simulink model "CarlaRosMatlab_LaneDetection"  (R2019b)
settings: Solver=FixedStepAuto  StartTime=0.0  StopTime=inf  FixedStep=0.2  RelTol=1e-3  EnableMultiTasking=on
model workspace (MAT data in the model file):
  SL_ROS_VariableLengthArrays_MaxSizes.CommonInfo.ArrayTruncateAction = 'EmitWarning'
  SL_ROS_VariableLengthArrays_MaxSizes.MsgTypeMap = containers.Map
  SL_ROS_VariableLengthArrays_MaxSizes.MsgTypeMap.serialization.keys = {'sensor_msgs/CompressedImage', 'sensor_msgs/Image', 'sensor_msgs/PointCloud2'}
  SL_ROS_VariableLengthArrays_MaxSizes.MsgTypeMap.serialization.values{1}(1).PropertyName = 'Format'
  SL_ROS_VariableLengthArrays_MaxSizes.MsgTypeMap.serialization.values{1}(1).DataType = 'uint8'
  SL_ROS_VariableLengthArrays_MaxSizes.MsgTypeMap.serialization.values{1}(1).MaxLength = 128
  SL_ROS_VariableLengthArrays_MaxSizes.MsgTypeMap.serialization.values{1}(2).PropertyName = 'Data'
  SL_ROS_VariableLengthArrays_MaxSizes.MsgTypeMap.serialization.values{1}(2).DataType = 'uint8'
  SL_ROS_VariableLengthArrays_MaxSizes.MsgTypeMap.serialization.values{1}(2).MaxLength = 128000
  SL_ROS_VariableLengthArrays_MaxSizes.MsgTypeMap.serialization.values{2}(1).PropertyName = 'Data'
  SL_ROS_VariableLengthArrays_MaxSizes.MsgTypeMap.serialization.values{2}(1).DataType = 'uint8'
  SL_ROS_VariableLengthArrays_MaxSizes.MsgTypeMap.serialization.values{2}(1).MaxLength = 8294400
  SL_ROS_VariableLengthArrays_MaxSizes.MsgTypeMap.serialization.values{2}(2).PropertyName = 'Encoding'
  SL_ROS_VariableLengthArrays_MaxSizes.MsgTypeMap.serialization.values{2}(2).DataType = 'uint8'
  SL_ROS_VariableLengthArrays_MaxSizes.MsgTypeMap.serialization.values{2}(2).MaxLength = 128
  SL_ROS_VariableLengthArrays_MaxSizes.MsgTypeMap.serialization.values{3}(1).PropertyName = 'Data'
  SL_ROS_VariableLengthArrays_MaxSizes.MsgTypeMap.serialization.values{3}(1).DataType = 'uint8'
  SL_ROS_VariableLengthArrays_MaxSizes.MsgTypeMap.serialization.values{3}(1).MaxLength = 182976
  SL_ROS_VariableLengthArrays_MaxSizes.MsgTypeMap.serialization.values{3}(2).PropertyName = 'Fields'
  SL_ROS_VariableLengthArrays_MaxSizes.MsgTypeMap.serialization.values{3}(2).DataType = 'sensor_msgs/PointField'
  SL_ROS_VariableLengthArrays_MaxSizes.MsgTypeMap.serialization.values{3}(2).MaxLength = 16
  SL_ROS_VariableLengthArrays_MaxSizes.MsgTypeMap.serialization.uniformity = 0
  SL_ROS_VariableLengthArrays_MaxSizes.MsgTypeMap.serialization.keyType = 'char'
  SL_ROS_VariableLengthArrays_MaxSizes.MsgTypeMap.serialization.valueType = 'any'
undefined symbols (not defined in the file or in its folder): Brake, Steer, Throttle
libraries: robotlib x10, visiontextngfix x2, visionsinks x2
settings Model: Creator=sprinkle  LastModifiedBy=aa
settings DataIOCC: ReturnWorkspaceOutputs=off
settings OptimizationCC: LifeSpan=Inf  MaxStackSize=64  EfficientTunableParamExpr=on
settings DebuggingCC: SFUnexpectedBacktrackingDiag=warning  SFNoUnconditionalDefaultTransitionDiag=warning  ArithmeticOperatorsInVariantConditions=warning
settings HardwareCC: ProdBitPerPointer=32  ProdBitPerSizeT=32  ProdBitPerPtrDiffT=32  ProdLargestAtomicFloat=None  ProdIntDivRoundTo=Undefined  ProdEndianess=Unspecified  ProdWordSize=32  ProdHWDeviceType=Generic->Unspecified (assume 32-bit Generic)
settings SFSimCC: SimUseLocalCustomCode=off  MATLABDynamicMemAlloc=off  CustomCodeUndefinedFunction=UseInterfaceOnly
settings RTWCC: SystemTargetFile=ert.tlc  HardwareBoard=Robot Operating System (ROS)  TLCOptions=-aInlineSetEventsForThisBaseRateFcn=TLC_FALSE -aSuppressMultiTaskScheduler=TLC_FALSE -aRateBasedStepFcn=0  TemplateMakefile=ert_default_tmf  GenerateReport=on  RTWUseLocalCustomCode=off  Toolchain=Catkin  IncludeHyperlinkInReport=on  LaunchReport=on  TargetLang=C++  GenerateTraceInfo=on  GenerateTraceReport=on  GenerateTraceReportSl=on  GenerateTraceReportSf=on  GenerateTraceReportEml=on
settings CodeAppCC: ForceParamTrailComments=on  IgnoreCustomStorageClasses=off  OperatorAnnotations=on  SimulinkDataObjDesc=on  SFDataObjDesc=on  MATLABFcnDesc=on  InsertBlockDesc=on  StateflowObjectComments=on  MATLABSourceComments=on
settings ERTTargetCC: MultiwordLength=2048
settings ConfigComp: CovMetricSettings=dw  CovHtmlReporting=on  CovSaveCumulativeToWorkspaceVar=on  CovSaveSingleToWorkspaceVar=on  CovExternalEMLEnable=off

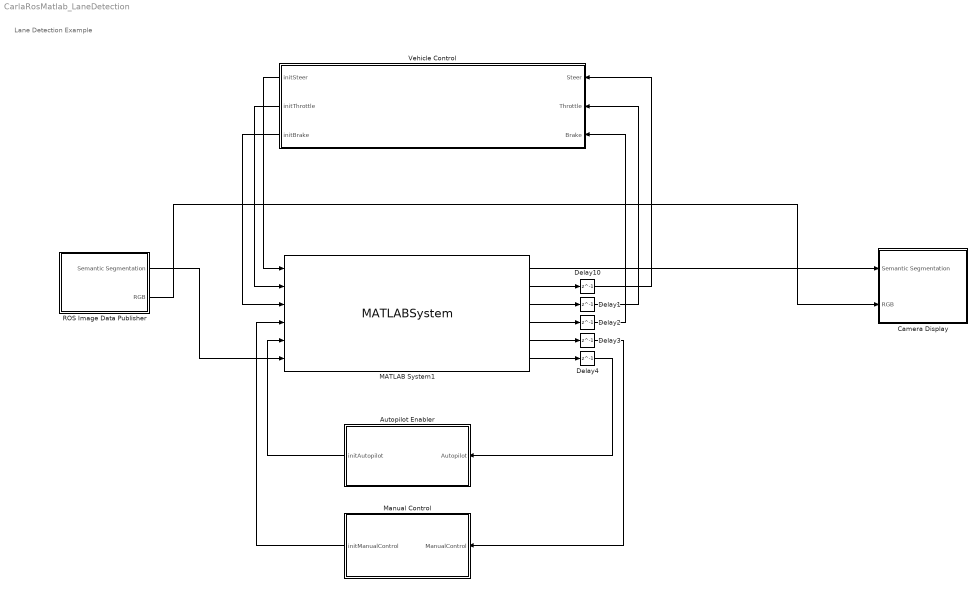
== system CarlaRosMatlab_LaneDetection ==
  note: Lane Detection Example
  Autopilot Enabler : Subsystem
  Camera Display : Subsystem
  Delay{1..4,10} (5 alike) : Delay  DelayLength=1  InitialCondition=0
  MATLAB System1 : MATLABSystem  System=LaneDetection  SimulateUsing=Interpreted execution
      mask Type: LaneDetection
      mask Display:
      | disp('LaneDetection');
      | port_label('input',1,'steer_prev');
      | port_label('input',2,'throttle_prev');
      | port_label('input',3,'brake_prev');
      | port_label('input',4,'manualcontrol_prev');
      | port_label('input',5,'autopilot_prev');
      | port_label('input',6,'SEMANTIC_IN');
      | port_label('output',1,'SEMANTIC_SEGMENTATION');
      | port_label('output',2,'steer');
      | port_label('output',3,'throttle');
      | port_label('output',4,'brake');
      | port_label('output',5,'manualcontrol');
      | port_label('output',6,'autopilot');
  Manual Control : Subsystem
  ROS Image Data Publisher : Subsystem
  Vehicle Control : Subsystem
  wires:
  MATLAB System1/1 -> Camera Display/1(Semantic Segmentation)
  ROS Image Data Publisher/2(RGB) -> Camera Display/2(RGB)
  Autopilot Enabler/1(initAutopilot) -> MATLAB System1/5
  Manual Control/1(initManualControl) -> MATLAB System1/4
  ROS Image Data Publisher/1(Semantic Segmentation) -> MATLAB System1/6
  MATLAB System1/2 -> Delay10/1
  MATLAB System1/3 -> Delay1/1
  MATLAB System1/4 -> Delay2/1
  MATLAB System1/5 -> Delay3/1
  MATLAB System1/6 -> Delay4/1
  Delay4/1 -> Autopilot Enabler/1(Autopilot)
  Delay3/1 -> Manual Control/1(ManualControl)
  Delay2/1 -> Vehicle Control/3(Brake)
  Delay1/1 -> Vehicle Control/2(Throttle)
  Vehicle Control/1(initSteer) -> MATLAB System1/1
  Vehicle Control/2(initThrottle) -> MATLAB System1/2
  Vehicle Control/3(initBrake) -> MATLAB System1/3
  Delay10/1 -> Vehicle Control/1(Steer)

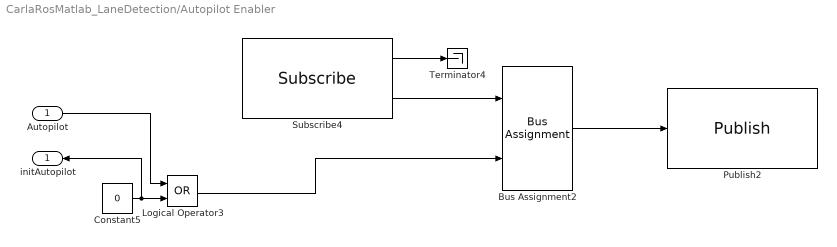
== system CarlaRosMatlab_LaneDetection/Autopilot Enabler ==
  Autopilot : Inport
  Bus Assignment2 : BusAssignment  AssignedSignals=Data
  Constant5 : Constant  Value=0  OutDataTypeStr=boolean
  Logical Operator3 : Logic  Operator=OR  AllPortsSameDT=off  OutDataTypeStr=boolean
  Publish2 : robotlib/Publish  topicSource=Select from ROS network  topic=/carla/ego_vehicle/enable_autopilot  messageType=std_msgs/Bool  messageQueueLength=1
      settings: SourceProductName=ROS Toolbox
  Subscribe4 : robotlib/Subscribe  topicSource=Select from ROS network  topic=/carla/ego_vehicle/enable_autopilot  messageType=std_msgs/Bool  sampleTime=-1  messageQueueLength=1
      settings: SourceProductName=ROS Toolbox
  Terminator4 : Terminator
  initAutopilot : Outport
  wires:
  Logical Operator3/1 -> Bus Assignment2/2
  Autopilot/1 -> Logical Operator3/1
  Bus Assignment2/1 -> Publish2/1
  Subscribe4/1 -> Terminator4/1
  Constant5/1 -> Logical Operator3/2, initAutopilot/1
  Subscribe4/2 -> Bus Assignment2/1

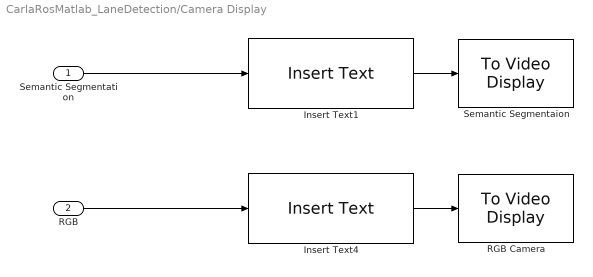
== system CarlaRosMatlab_LaneDetection/Camera Display ==
  Semantic Segmentation : Inport
  RGB : Inport  Port=2
  Insert Text1 : visiontextngfix/Insert Text  inputType=Obsolete  theText='Carla Ros Bridge Semantic Segmentation'  getTextLocFrom=Specify via dialog  textLoc=[1 1]  getTextColorFrom=Specify via dialog  textColor=[0 0 0]  getTextIntensityFrom=Specify via dialog  textIntensity=0  getTextOpacityFrom=Specify via dialog  textOpacity=1.0  dummyVar2=0  dummyVar3=0  dummyVar4=0  imagePorts=One multidimensional signal  isInputTransposed=off  fontFace=LucidaSansRegular  dummyVar1=0  blockFontSize=24  antiAliased=on
      settings: SourceProductName=Computer Vision Toolbox  SourceProductBaseCode=VP
  Insert Text4 : visiontextngfix/Insert Text  inputType=Obsolete  theText='Carla Ros Bridge RGB Camera'  getTextLocFrom=Specify via dialog  textLoc=[1 1]  getTextColorFrom=Specify via dialog  textColor=[0 0 0]  getTextIntensityFrom=Specify via dialog  textIntensity=0  getTextOpacityFrom=Specify via dialog  textOpacity=1.0  dummyVar2=0  dummyVar3=0  dummyVar4=0  imagePorts=One multidimensional signal  isInputTransposed=off  fontFace=LucidaSansRegular  dummyVar1=0  blockFontSize=24  antiAliased=on
      settings: SourceProductName=Computer Vision Toolbox  SourceProductBaseCode=VP
  RGB Camera : visionsinks/To Video Display  windowSizeMode=Normal  openAtMdlStart=on  fullScreen=off  videoWindowX=2846  videoWindowY=146  saveWindowSize=off  videoWindowWidth=928  videoWindowHeight=1028  inputColorFormat=RGB  inputType=Obsolete  imagePorts=One multidimensional signal  OutputDevice=On-screen video monitor  dataOrg=Column-major  isWindowOpen=off
      settings: SourceProductName=Computer Vision Toolbox
  Semantic Segmentaion : visionsinks/To Video Display  windowSizeMode=Normal  openAtMdlStart=on  fullScreen=off  videoWindowX=2036  videoWindowY=308  saveWindowSize=off  videoWindowWidth=960  videoWindowHeight=534  inputColorFormat=RGB  inputType=Obsolete  imagePorts=One multidimensional signal  OutputDevice=On-screen video monitor  dataOrg=Column-major  isWindowOpen=off
      settings: SourceProductName=Computer Vision Toolbox
  wires:
  Insert Text4/1 -> RGB Camera/1
  Semantic Segmentation/1 -> Insert Text1/1
  Insert Text1/1 -> Semantic Segmentaion/1
  RGB/1 -> Insert Text4/1

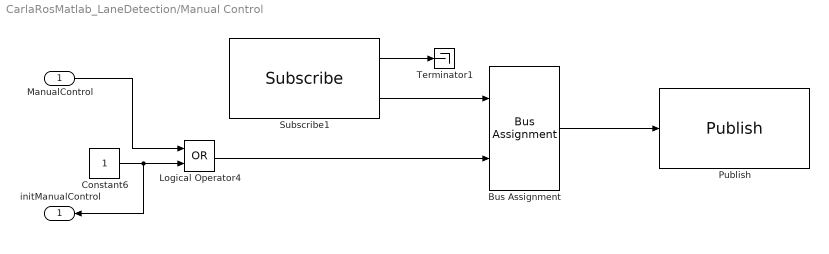
== system CarlaRosMatlab_LaneDetection/Manual Control ==
  ManualControl : Inport
  Bus Assignment : BusAssignment  AssignedSignals=Data
  Constant6 : Constant  OutDataTypeStr=boolean
  Logical Operator4 : Logic  Operator=OR  AllPortsSameDT=off  OutDataTypeStr=boolean
  Publish : robotlib/Publish  topicSource=Select from ROS network  topic=/carla/ego_vehicle/vehicle_control_manual_override  messageType=std_msgs/Bool  messageQueueLength=1
      settings: SourceProductName=ROS Toolbox
  Subscribe1 : robotlib/Subscribe  topicSource=Select from ROS network  topic=/carla/ego_vehicle/vehicle_control_manual_override  messageType=std_msgs/Bool  sampleTime=-1  messageQueueLength=1
      settings: SourceProductName=ROS Toolbox
  Terminator1 : Terminator
  initManualControl : Outport
  wires:
  Constant6/1 -> Logical Operator4/2, initManualControl/1
  Subscribe1/1 -> Terminator1/1
  Logical Operator4/1 -> Bus Assignment/2
  ManualControl/1 -> Logical Operator4/1
  Bus Assignment/1 -> Publish/1
  Subscribe1/2 -> Bus Assignment/1

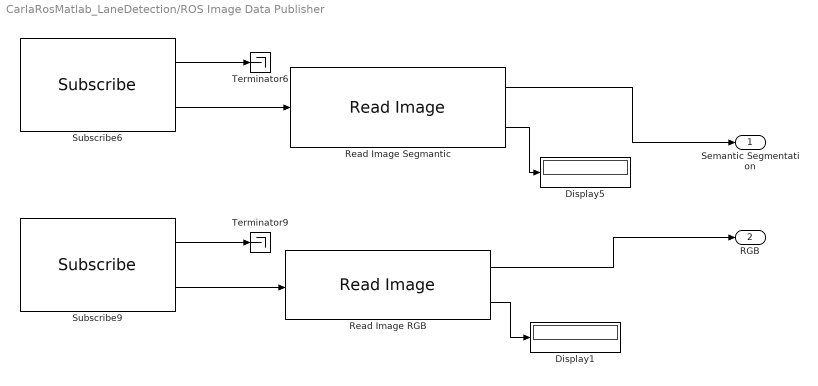
== system CarlaRosMatlab_LaneDetection/ROS Image Data Publisher ==
  Display1 : Display
  Display5 : Display
  Read Image RGB : robotlib/Read Image  MaximumImageSize=[600, 800]  ImageEncoding=bgra8  ShowAlphaOutput=off  ShowErrorCodeOutput=on  VariableSizeOutputs=on
      settings: SourceProductName=Robotics System Toolbox  SourceProductBaseCode=RO
  Read Image Segmantic : robotlib/Read Image  MaximumImageSize=[540, 960]  ImageEncoding=bgra8  ShowAlphaOutput=off  ShowErrorCodeOutput=on  VariableSizeOutputs=on
      settings: SourceProductName=ROS Toolbox  SourceProductBaseCode=RR
  Subscribe6 : robotlib/Subscribe  topicSource=Select from ROS network  topic=/carla/ego_vehicle/camera/semantic_segmentation/fronts/image_segmentation  messageType=sensor_msgs/Image  sampleTime=-1  messageQueueLength=1
      settings: SourceProductBaseCode=RO
  Subscribe9 : robotlib/Subscribe  topicSource=Select from ROS network  topic=/carla/ego_vehicle/camera/rgb/front/image_color  messageType=sensor_msgs/Image  sampleTime=-1  messageQueueLength=1
      settings: SourceProductBaseCode=RO
  Terminator6 : Terminator
  Terminator9 : Terminator
  Semantic Segmentation : Outport
  RGB : Outport  Port=2
  wires:
  Subscribe6/1 -> Terminator6/1
  Read Image Segmantic/1 -> Semantic Segmentation/1
  Subscribe9/1 -> Terminator9/1
  Read Image RGB/1 -> RGB/1
  Subscribe9/2 -> Read Image RGB/1
  Read Image Segmantic/2 -> Display5/1
  Subscribe6/2 -> Read Image Segmantic/1
  Read Image RGB/2 -> Display1/1

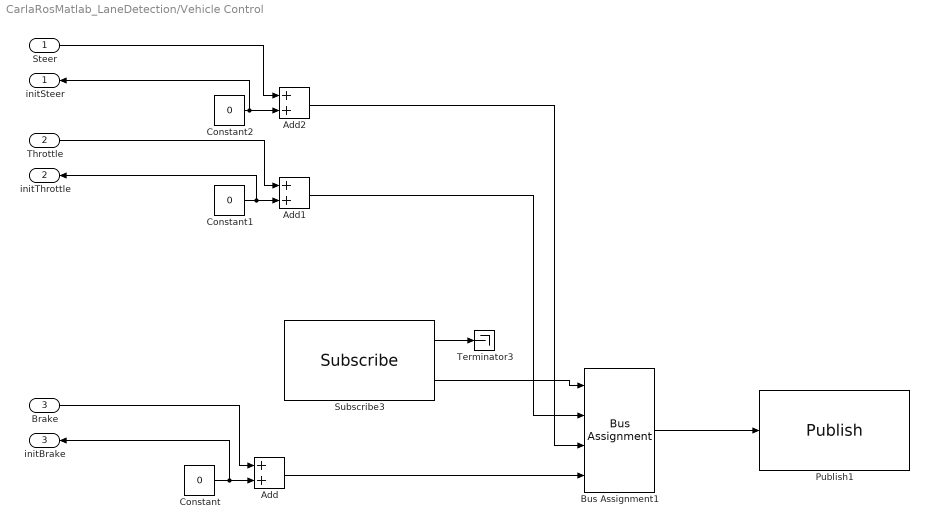
== system CarlaRosMatlab_LaneDetection/Vehicle Control ==
  Steer : Inport
  Throttle : Inport  Port=2
  Brake : Inport  Port=3
  Add : Sum
  Add1 : Sum
  Add2 : Sum
  Bus Assignment1 : BusAssignment  AssignedSignals=Throttle,Steer,Brake
  Constant : Constant  Value=0  OutDataTypeStr=single
  Constant1 : Constant  Value=0  OutDataTypeStr=single
  Constant2 : Constant  Value=0  OutDataTypeStr=single
  Publish1 : robotlib/Publish  topicSource=Select from ROS network  topic=/carla/ego_vehicle/vehicle_control_cmd_manual  messageType=carla_msgs/CarlaEgoVehicleControl  messageQueueLength=1
      settings: SourceProductName=ROS Toolbox
  Subscribe3 : robotlib/Subscribe  topicSource=Select from ROS network  topic=/carla/ego_vehicle/vehicle_control_cmd_manual  messageType=carla_msgs/CarlaEgoVehicleControl  sampleTime=-1  messageQueueLength=1
      settings: SourceProductName=ROS Toolbox
  Terminator3 : Terminator
  initSteer : Outport
  initThrottle : Outport  Port=2
  initBrake : Outport  Port=3
  wires:
  Steer/1 -> Add2/1
  Constant2/1 -> initSteer/1, Add2/2
  Throttle/1 -> Add1/1
  Constant1/1 -> initThrottle/1, Add1/2
  Constant/1 -> initBrake/1, Add/2
  Brake/1 -> Add/1
  Add1/1 -> Bus Assignment1/2
  Subscribe3/1 -> Terminator3/1
  Subscribe3/2 -> Bus Assignment1/1
  Add2/1 -> Bus Assignment1/3
  Bus Assignment1/1 -> Publish1/1
  Add/1 -> Bus Assignment1/4
